simulink model "Simulation_model_side_A"  (R2021a)
settings: Solver=ode23t  StartTime=0.0  StopTime=6  FixedStep=T  RelTol=1e-3
values from neighbouring files (symbols this model uses):
  C_dc = Cb*c_dc_pu    [parameters.m]
  C_f = Cb*c_f_pu    [parameters.m]
  f_SM = fb    (= 50)    [parameters.m]
  fb = 50    [parameters.m]
  ff_SM = 0.01322    [parameters.m]
  Ib = 2/3*Sb/Vb    [parameters.m]
  Ib_dc = Sb/Vb_dc    [parameters.m]
  ic_SM = 0.8    [parameters.m]
  K_ad = 1.5    [parameters.m]
  K_ffv = 0    [parameters.m]
  K_ic = K_pc/T_1    [parameters.m]
  K_idc = K_pdc/T_idc    (= 250)    [parameters.m]
  K_iPLL = a^2*T_fPLL    (= 0.09)    [parameters.m]
  K_iv = K_pv/T_iv    (= 92.0050761421)    [parameters.m]
  K_iv_SM = K_pv_SM/T_iv_SM    (= 70)    [parameters.m]
  K_omega = 20    [parameters.m]
  K_omega_SM = 40    [parameters.m]
  K_pc = l_f_pu/(4*pi*fb*T_sum)    (= 1.27323954474)    [parameters.m]
  K_pdc = 25    [parameters.m]
  K_pPLL = 1/(a*2*pi*T_fPLL)    (= 5.30516476973)    [parameters.m]
  K_pv = 0.29    [parameters.m]
  K_pv_SM = 35    [parameters.m]
  K_vco = 2*pi    (= 6.28318530718)    [parameters.m]
  Kd = 40    [parameters.m]
  Kq = 0.1    [parameters.m]
  Kq_SM = 0.1    [parameters.m]
  L_f = Lb*l_f_pu    [parameters.m]
  l_f_pu = 0.08    [parameters.m]
  lf1f = 0    [parameters.m]
  lfd_SM = 0.531    [parameters.m]
  llkd = 2.655    [parameters.m]
  llkq1 = 0.2408    [parameters.m]
  lls_SM = 0.08    [parameters.m]
  lmd_SM = 2.81    [parameters.m]
  lmq_SM = 1.64    [parameters.m]
  omega_ad = 50    [parameters.m]
  omega_b = 2*pi*fb    (= 314.159265359)    [parameters.m]
  omega_d = 5    [parameters.m]
  omega_qf = 200    [parameters.m]
  omega_qf_SM = 200    [parameters.m]
  omega_vf = 200    [parameters.m]
  p_h = 0.1    [parameters.m]
  pp_SM = 2    [parameters.m]
  R_lf = Rb*r_lf_pu    [parameters.m]
  rfd_SM = 0.004319    [parameters.m]
  rkd = 0.2343    [parameters.m]
  rkq1 = 0.03365    [parameters.m]
  rs_SM = 0.01524    [parameters.m]
  S_SM = Sb    (= 1000000)    [parameters.m]
  Sb = 1e6    (= 1000000)    [parameters.m]
  T = 1e-4    (= 0.0001)    [parameters.m]
  T_fPLL = 10e-3    (= 0.01)    [parameters.m]
  T_gt_SM = 0.5    [parameters.m]
  Ta = 4    [parameters.m]
  v_dc_ref = 1    [parameters.m]
  V_SM = V    (= 690)    [parameters.m]
  Vb = V*sqrt(2)/sqrt(3)    [parameters.m]
  Vb_dc = Vb*2    [parameters.m]
undefined symbols (not defined in the file or in its folder): D11, Delta
libraries: simulink_extras x18, spsDiodeLib x12, spsThreePhaseVIMeasurementLib x9, spsThreePhaseSeriesRLCBranchLib x7, spsPower3phInstantaneousLib x5, spsVoltageMeasurementLib x3, spsControlledCurrentSourceLib x2, spsThreePhaseParallelRLCLoadLib x2, spsThreePhaseBreakerLib x2, spsUniversalBridgeLib x2, spsDCVoltageSourceLib x1, spsGroundLib x1
(part 2 of 2)

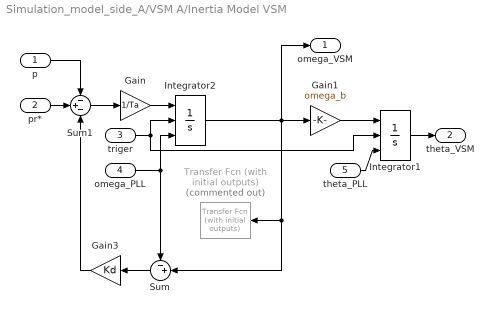
== system Simulation_model_side_A/VSM A/Inertia Model VSM ==
  p : Inport
  pr* : Inport  Port=2
  triger : Inport  Port=3
  omega_PLL : Inport  Port=4
  theta_PLL : Inport  Port=5
  Gain : Gain  Gain=1/Ta
  Gain1 : Gain  Gain=omega_b
  Gain3 : Gain  Gain=Kd
  Integrator1 : Integrator  ExternalReset=level hold  InitialConditionSource=external  InitialCondition=1  WrapState=on  WrappedStateUpperValue=2*pi  WrappedStateLowerValue=0
  Integrator2 : Integrator  ExternalReset=level hold  InitialConditionSource=external  InitialCondition=1
  Sum : Sum  Inputs=-+|
  Sum1 : Sum  Inputs=-+-
  Transfer Fcn (with initial outputs) : simulink_extras/Additional Linear/Transfer Fcn (with initial outputs)  Commented=on  N=[omega_d]  D="[1  omega_d]"  Y0=1  U0=1
  omega_VSM : Outport
  theta_VSM : Outport  Port=2
  wires:
  Gain/1 -> Integrator2/1
  Gain3/1 -> Sum1/3
  Sum1/1 -> Gain/1
  p/1 -> Sum1/1
  pr*/1 -> Sum1/2
  Integrator1/1 -> theta_VSM/1
  Integrator2/1 -> Sum/2, Transfer Fcn (with initial outputs)/1, Gain1/1, omega_VSM/1
  theta_PLL/1 -> Integrator1/3
  triger/1 -> Integrator2/2, Integrator1/2
  Gain1/1 -> Integrator1/1
  omega_PLL/1 -> Integrator2/3, Sum/1
  Sum/1 -> Gain3/1

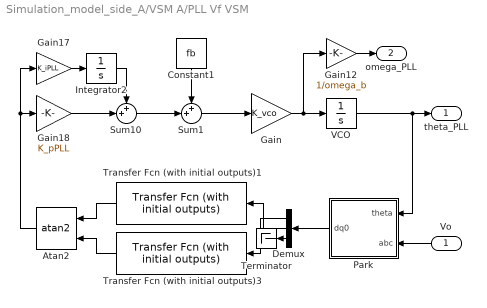
== system Simulation_model_side_A/VSM A/PLL Vf VSM ==
  Vo : Inport
  Atan2 : Trigonometry  Operator=atan2  OutputSignalType=real
  Constant1 : Constant  Value=fb
  Demux : Demux  Outputs=3
  Gain : Gain  Gain=K_vco
  Gain12 : Gain  Gain=1/omega_b
  Gain17 : Gain  Gain=K_iPLL
  Gain18 : Gain  Gain=K_pPLL
  Integrator2 : Integrator
  Park : MATLAB Function  TreatAsAtomicUnit=on
  Sum1 : Sum  Inputs=++|
  Sum10 : Sum  Inputs=++|
  Terminator : Terminator
  Transfer Fcn (with initial outputs)1 : simulink_extras/Additional Linear/Transfer Fcn (with initial outputs)  N=[1]  D=[T_fPLL, 1]  Y0=0  U0=0
  Transfer Fcn (with initial outputs)3 : simulink_extras/Additional Linear/Transfer Fcn (with initial outputs)  N=[1]  D=[T_fPLL, 1]  Y0=1  U0=1
  VCO : Integrator  WrapState=on  WrappedStateUpperValue=2*pi  WrappedStateLowerValue=0
  theta_PLL : Outport
  omega_PLL : Outport  Port=2
  wires:
  Transfer Fcn (with initial outputs)1/1 -> Atan2/1
  Transfer Fcn (with initial outputs)3/1 -> Atan2/2
  VCO/1 -> theta_PLL/1, Park/1(theta)
  Sum1/1 -> Gain/1
  Gain/1 -> Gain12/1, VCO/1
  Constant1/1 -> Sum1/1
  Park/1(dq0) -> Demux/1
  Sum10/1 -> Sum1/2
  Atan2/1 -> Gain18/1, Gain17/1
  Demux/1 -> Transfer Fcn (with initial outputs)3/1
  Demux/2 -> Transfer Fcn (with initial outputs)1/1
  Vo/1 -> Park/2(abc)
  Gain18/1 -> Sum10/2
  Integrator2/1 -> Sum10/1
  Gain17/1 -> Integrator2/1
  Gain12/1 -> omega_PLL/1
  Demux/3 -> Terminator/1

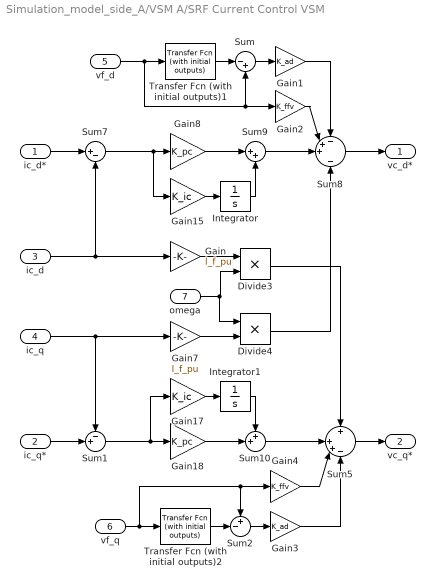
== system Simulation_model_side_A/VSM A/SRF Current Control VSM ==
  ic_d* : Inport
  ic_q* : Inport  Port=2
  ic_d : Inport  Port=3
  ic_q : Inport  Port=4
  vf_d : Inport  Port=5
  vf_q : Inport  Port=6
  omega : Inport  Port=7
  Divide3 : Product  Inputs=**
  Divide4 : Product  Inputs=**
  Gain : Gain  Gain=l_f_pu
  Gain1 : Gain  Gain=K_ad
  Gain15 : Gain  Gain=K_ic
  Gain17 : Gain  Gain=K_ic
  Gain18 : Gain  Gain=K_pc
  Gain2 : Gain  Gain=K_ffv
  Gain3 : Gain  Gain=K_ad
  Gain4 : Gain  Gain=K_ffv
  Gain7 : Gain  Gain=l_f_pu
  Gain8 : Gain  Gain=K_pc
  Integrator : Integrator  InitialCondition=1
  Integrator1 : Integrator
  Sum : Sum  Inputs=|-+
  Sum1 : Sum  Inputs=-+|
  Sum10 : Sum  Inputs=++|
  Sum2 : Sum  Inputs=+-|
  Sum5 : Sum  Inputs=+|++-
  Sum7 : Sum  Inputs=|+-
  Sum8 : Sum  Inputs=-++|-
  Sum9 : Sum  Inputs=|++
  Transfer Fcn (with initial outputs)1 : simulink_extras/Additional Linear/Transfer Fcn (with initial outputs)  N=[omega_ad]  D="[1  omega_ad]"  Y0=1  U0=1
  Transfer Fcn (with initial outputs)2 : simulink_extras/Additional Linear/Transfer Fcn (with initial outputs)  N=[omega_ad]  D="[1  omega_ad]"  Y0=0  U0=0
  vc_d* : Outport
  vc_q* : Outport  Port=2
  wires:
  ic_q*/1 -> Sum1/2
  Sum7/1 -> Gain15/1, Gain8/1
  Gain15/1 -> Integrator/1
  Sum1/1 -> Gain18/1, Gain17/1
  Divide3/1 -> Sum5/1
  Divide4/1 -> Sum8/4
  Gain7/1 -> Divide4/2
  Gain/1 -> Divide3/1
  Gain17/1 -> Integrator1/1
  Sum9/1 -> Sum8/3
  Integrator1/1 -> Sum10/1
  omega/1 -> Divide4/1, Divide3/2
  Gain18/1 -> Sum10/2
  Sum8/1 -> vc_d*/1
  Sum10/1 -> Sum5/2
  Gain8/1 -> Sum9/1
  ic_q/1 -> Gain7/1, Sum1/1
  Integrator/1 -> Sum9/2
  ic_d/1 -> Gain/1, Sum7/2
  ic_d*/1 -> Sum7/1
  Sum5/1 -> vc_q*/1
  Transfer Fcn (with initial outputs)1/1 -> Sum/1
  Sum/1 -> Gain1/1
  Gain1/1 -> Sum8/1
  vf_d/1 -> Transfer Fcn (with initial outputs)1/1, Sum/2, Gain2/1
  Gain2/1 -> Sum8/2
  Sum2/1 -> Gain3/1
  vf_q/1 -> Sum2/1, Gain4/1, Transfer Fcn (with initial outputs)2/1
  Transfer Fcn (with initial outputs)2/1 -> Sum2/2
  Gain4/1 -> Sum5/3
  Gain3/1 -> Sum5/4

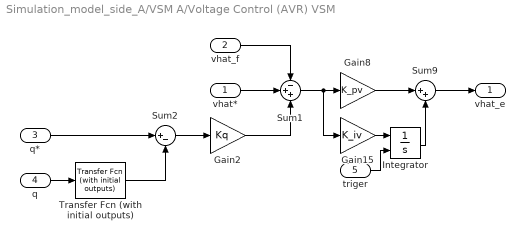
== system Simulation_model_side_A/VSM A/Voltage Control (AVR) VSM ==
  vhat* : Inport
  vhat_f : Inport  Port=2
  q* : Inport  Port=3
  q : Inport  Port=4
  triger : Inport  Port=5
  Gain15 : Gain  Gain=K_iv
  Gain2 : Gain  Gain=Kq
  Gain8 : Gain  Gain=K_pv
  Integrator : Integrator  ExternalReset=level hold
  Sum1 : Sum  Inputs=-++
  Sum2 : Sum  Inputs=|+-
  Sum9 : Sum  Inputs=|++
  Transfer Fcn (with initial outputs) : simulink_extras/Additional Linear/Transfer Fcn (with initial outputs)  N=[omega_qf]  D="[1  omega_qf]"  Y0=0  U0=0
  vhat_e : Outport
  wires:
  Sum9/1 -> vhat_e/1
  Integrator/1 -> Sum9/2
  Sum1/1 -> Gain15/1, Gain8/1
  Gain15/1 -> Integrator/1
  Gain8/1 -> Sum9/1
  vhat_f/1 -> Sum1/1
  q*/1 -> Sum2/1
  q/1 -> Transfer Fcn (with initial outputs)/1
  Transfer Fcn (with initial outputs)/1 -> Sum2/2
  Sum2/1 -> Gain2/1
  vhat*/1 -> Sum1/2
  Gain2/1 -> Sum1/3
  triger/1 -> Integrator/2

== matlab function Simulation_model_side_A/VSM A/abs vhat_f VSM ==
  data: vd input; v_abs output; vq input
function v_abs = abs(vd, vq)
% clark trasformation

v_abs = sqrt(vd^2+vq^2);

== matlab function Simulation_model_side_A/VSC Load A/PLL VSC/Park ==
  data: wt input; abc input; dq0 output
function dq0 = Park(wt, abc)
% Park trasformation
dq0 = 2/3*[cos(wt),  cos(wt-(2*pi/3)),  cos(wt+(2*pi/3));
          -sin(wt), -sin(wt-(2*pi/3)), -sin(wt+(2*pi/3));
               1/2,               1/2,               1/2]*abc;

== matlab function Simulation_model_side_A/VSC Load A/Park Ic VSC ==
  data: abc input; wt input; dq0 output
function dq0 = Park(abc, wt)
% Park trasformation
dq0 = 2/3*[cos(wt),  cos(wt-(2*pi/3)),  cos(wt+(2*pi/3));
          -sin(wt), -sin(wt-(2*pi/3)), -sin(wt+(2*pi/3));
               1/2,               1/2,               1/2]*abc;

== matlab function Simulation_model_side_A/VSC Load A/Park Vf VSC ==
  data: abc input; wt input; dq0 output
function dq0 = Park(abc, wt)
% Park trasformation
dq0 = 2/3*[cos(wt),  cos(wt-(2*pi/3)),  cos(wt+(2*pi/3));
          -sin(wt), -sin(wt-(2*pi/3)), -sin(wt+(2*pi/3));
               1/2,               1/2,               1/2]*abc;

== matlab function Simulation_model_side_A/VSC Load A/Power calk VSC ==
  data: vd input; vq input; p output; q output; id input; iq input
function [p, q]= PQ_Calk(vd, vq, id, iq)
% clark trasformation


p = vd*id + vq*iq;
q = -vd*iq + vq*id;

== matlab function Simulation_model_side_A/PLL grid/Park ==
  data: theta input; abc input; dq0 output
function dq0 = Park(theta, abc)
% Park trasformation
dq0 = 2/3*[cos(theta),  cos(theta-(2*pi/3)),  cos(theta+(2*pi/3));
          -sin(theta), -sin(theta-(2*pi/3)), -sin(theta+(2*pi/3));
               1/2,               1/2,               1/2]*abc;

== matlab function Simulation_model_side_A/PLL grid/abs vhat_f VSM ==
  data: vd input; v_abs output; vq input
function v_abs = abs(vd, vq)
% clark trasformation

v_abs = sqrt(vd^2+vq^2);

== matlab function Simulation_model_side_A/VSC Load A/"PWM" with 3 harmonic VSC/inv Park ==
  data: dq0 input; wt input; abc output
function abc = inv_Park(dq0, wt)
% Park trasformation
abc = [         cos(wt),          -sin(wt), 1;
       cos(wt-(2*pi/3)), -sin(wt-(2*pi/3)), 1;
       cos(wt+(2*pi/3)), -sin(wt+(2*pi/3)), 1]*dq0;

== matlab function Simulation_model_side_A/VSM A/"PWM" with 3 harmonic VSM/inv Park ==
  data: dq0 input; wt input; abc output
function abc = inv_Park(dq0, wt)
% Park trasformation
abc = [         cos(wt),          -sin(wt), 1;
       cos(wt-(2*pi/3)), -sin(wt-(2*pi/3)), 1;
       cos(wt+(2*pi/3)), -sin(wt+(2*pi/3)), 1]*dq0;

== matlab function Simulation_model_side_A/VSM A/Electrical Model VSM ==
  data: vhat_e input; omega input; vmd input; id_star output; iq_star output; vmq input; triger input
function [id_star, iq_star] = Electrical_model(vhat_e, omega, vmd, vmq, triger)
% Electrical model of the syncronus machine.  

rs = 0.01;    % Internal resistans of the VSM [pu]
ls = 0.25;    % Internal inductance of the VSM [pu]

if triger == 1
id_star = 0;
iq_star = 0;      
else
id_star = (rs * (vhat_e - vmd))/(rs^2+(ls*omega)^2)  - ((ls*omega)*vmq)/(rs^2+(ls*omega)^2);
iq_star = -(rs * vmq)/(rs^2+(ls*omega)^2) - ((ls*omega)*(vhat_e - vmd))/(rs^2+(ls*omega)^2);
end

== matlab function Simulation_model_side_A/VSM A/PLL Vf VSM/Park ==
  data: theta input; abc input; dq0 output
function dq0 = Park(theta, abc)
% Park trasformation
dq0 = 2/3*[cos(theta),  cos(theta-(2*pi/3)),  cos(theta+(2*pi/3));
          -sin(theta), -sin(theta-(2*pi/3)), -sin(theta+(2*pi/3));
               1/2,               1/2,               1/2]*abc;

== matlab function Simulation_model_side_A/VSM A/PQ calk VSM ==
  data: vd input; vq input; p output; q output; id input; iq input
function [p, q]= PQ_Calk(vd, vq, id, iq)
% clark trasformation

p = vd*id + vq*iq;
q = -vd*iq + vq*id;

== matlab function Simulation_model_side_A/abs(v_hat) SM A ==
  data: vd input; v_abs output; vq input
function v_abs = abs(vd, vq)
% clark trasformation

v_abs = sqrt(vd^2+vq^2);

== matlab function Simulation_model_side_A/VSM A/Park Ic VSM ==
  data: abc input; theta input; dq0 output
function dq0 = Park(abc, theta)
% Park trasformation
dq0 = 2/3*[cos(theta),  cos(theta-(2*pi/3)),  cos(theta+(2*pi/3));
          -sin(theta), -sin(theta-(2*pi/3)), -sin(theta+(2*pi/3));
               1/2,               1/2,               1/2]*abc;

== matlab function Simulation_model_side_A/VSM A/Park Vf VSM ==
  data: abc input; theta input; dq0 output
function dq0 = Park(abc, theta)
% Park trasformation
dq0 = 2/3*[cos(theta),  cos(theta-(2*pi/3)),  cos(theta+(2*pi/3));
          -sin(theta), -sin(theta-(2*pi/3)), -sin(theta+(2*pi/3));
               1/2,               1/2,               1/2]*abc;
